simulink model "ELECTRIC_CIRCUIT_FINAL"  (R2018b)
settings: Solver=VariableStepAuto  StartTime=0.0  StopTime=6*10^-5  RelTol=1e-3
libraries: fl_lib x23, nesl_utility x14
settings Model: Creator=EmanuelCruvinel  LastModifiedBy=EmanuelCruvinel
settings SimscapeCC: SimscapeLogType=all

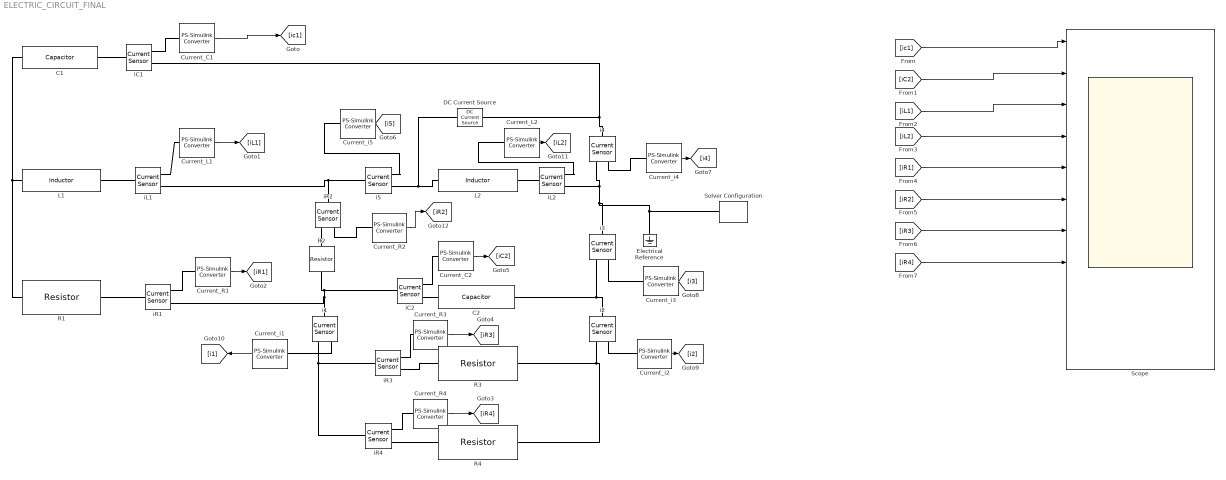
== system ELECTRIC_CIRCUIT_FINAL ==
  C1 : fl_lib/Electrical/Electrical Elements/Capacitor  c=1e-6 F  r=1e-6 Ohm  g=0 1/Ohm  i_specify=off  i_priority=None  i=0 A  i_nominal_specify=off  i_nominal_unit=A  i_nominal_value=1  v_specify=off  v_priority=None  v=0 V  v_nominal_specify=off  v_nominal_unit=V  v_nominal_value=1  vc_specify=off  vc_priority=High  vc=0 V  vc_nominal_specify=off  vc_nominal_unit=V  vc_nominal_value=1
  C2 : fl_lib/Electrical/Electrical Elements/Capacitor  c=1e-6 F  r=1e-6 Ohm  g=0 1/Ohm  i_specify=off  i_priority=None  i=0 A  i_nominal_specify=off  i_nominal_unit=A  i_nominal_value=1  v_specify=off  v_priority=None  v=0 V  v_nominal_specify=off  v_nominal_unit=V  v_nominal_value=1  vc_specify=off  vc_priority=High  vc=0 V  vc_nominal_specify=off  vc_nominal_unit=V  vc_nominal_value=1
  Current_C1 : nesl_utility/PS-Simulink Converter  PhysicalDomain=network_engine_domain  SubClassName=ps_output  LeftPortType=input  RightPortType=output  PseudoPeriodic=off  Frequencies=[]  Unit=1  AffineConversion=off
  Current_C2 : nesl_utility/PS-Simulink Converter  PhysicalDomain=network_engine_domain  SubClassName=ps_output  LeftPortType=input  RightPortType=output  PseudoPeriodic=off  Frequencies=[]  Unit=1  AffineConversion=off
  Current_L1 : nesl_utility/PS-Simulink Converter  PhysicalDomain=network_engine_domain  SubClassName=ps_output  LeftPortType=input  RightPortType=output  PseudoPeriodic=off  Frequencies=[]  Unit=1  AffineConversion=off
  Current_L2 : nesl_utility/PS-Simulink Converter  PhysicalDomain=network_engine_domain  SubClassName=ps_output  LeftPortType=input  RightPortType=output  PseudoPeriodic=off  Frequencies=[]  Unit=1  AffineConversion=off
  Current_R{1..4} (4 alike) : nesl_utility/PS-Simulink Converter  PhysicalDomain=network_engine_domain  SubClassName=ps_output  LeftPortType=input  RightPortType=output  PseudoPeriodic=off  Frequencies=[]  Unit=1  AffineConversion=off
  Current_i{1..5} (5 alike) : nesl_utility/PS-Simulink Converter  PhysicalDomain=network_engine_domain  SubClassName=ps_output  LeftPortType=input  RightPortType=output  PseudoPeriodic=off  Frequencies=[]  Unit=1  AffineConversion=off
  DC Current Source : fl_lib/Electrical/Electrical Sources/DC Current Source  i0=200 A
      settings: SourceProductName=Simscape  SourceProductBaseCode=SS
  Electrical Reference : fl_lib/Electrical/Electrical Elements/Electrical Reference
  L1 : fl_lib/Electrical/Electrical Elements/Inductor  l=1e-6 H  r=0 Ohm  g=1e-9 1/Ohm  i_specify=off  i_priority=None  i=0 A  i_nominal_specify=off  i_nominal_unit=A  i_nominal_value=1  v_specify=off  v_priority=None  v=0 V  v_nominal_specify=off  v_nominal_unit=V  v_nominal_value=1  i_L_specify=off  i_L_priority=High  i_L=0 A  i_L_nominal_specify=off  i_L_nominal_unit=A  i_L_nominal_value=1
  L2 : fl_lib/Electrical/Electrical Elements/Inductor  l=1e-6 H  r=0 Ohm  g=1e-9 1/Ohm  i_specify=off  i_priority=None  i=0 A  i_nominal_specify=off  i_nominal_unit=A  i_nominal_value=1  v_specify=off  v_priority=None  v=0 V  v_nominal_specify=off  v_nominal_unit=V  v_nominal_value=1  i_L_specify=off  i_L_priority=High  i_L=0 A  i_L_nominal_specify=off  i_L_nominal_unit=A  i_L_nominal_value=1
  R{1..4} (4 alike) : fl_lib/Electrical/Electrical Elements/Resistor  R=10 Ohm  i_specify=off  i_priority=None  i=0 A  i_nominal_specify=off  i_nominal_unit=A  i_nominal_value=1  v_specify=off  v_priority=None  v=0 V  v_nominal_specify=off  v_nominal_unit=V  v_nominal_value=1
      R1 settings: LogSimulationData=on
  Scope : Scope  NumInputPorts=11
  Solver Configuration : nesl_utility/Solver Configuration  PhysicalDomain=network_engine_domain  SubClassName=solver  LeftPortType=input  RightPortType=generic  Tones=[]  Harmonics=[]  SimulateNoise=off  Profile=off  UseLocalSampling=off  EnableSwitchedLinearOptims=on  FrequencyDomain=off  UseCCode=off  RelTol=0.001  AbsTol=1e-06  MinStep=1e-09  ToWorkspace=off  RevertToSquareIcSolve=off  NumHomotopyIterations=100  PhasorMode=off  PhasorModeNumHarmonics=1  DoDC=off  ResidualTolerance=1e-09  UseLocalSolver=off  LocalSolverChoice=NE_BACKWARD_EULER_ADVANCER  LocalSolverSampleTime=0.001  DoFixedCost=off  MaxNonlinIter=3  MaxModeIter=2  LinearAlgebra=auto  EquationFormulation=NE_TIME_EF  DelaysMemoryBudget=1024  AutomaticFiltering=on  FilteringTimeConstant=0.001  PartitionStorageMethod=AS_NEEDED  PartitionMemoryBudget=1024
  i{1..5} (5 alike) : fl_lib/Electrical/Electrical Sensors/Current Sensor
  iC1 : fl_lib/Electrical/Electrical Sensors/Current Sensor
  iC2 : fl_lib/Electrical/Electrical Sensors/Current Sensor
  iL1 : fl_lib/Electrical/Electrical Sensors/Current Sensor
  iL2 : fl_lib/Electrical/Electrical Sensors/Current Sensor
  iR{1..4} (4 alike) : fl_lib/Electrical/Electrical Sensors/Current Sensor
  wires:
  Current_C1/1 -> [ic1]
  [ic1] -> Scope/1
  Current_L1/1 -> [iL1]
  Current_R1/1 -> [iR1]
  Current_R4/1 -> [iR4]
  Current_R3/1 -> [iR3]
  Current_C2/1 -> [iC2]
  Current_i5/1 -> [i5]
  Current_i4/1 -> [i4]
  Current_i2/1 -> [i2]
  Current_i1/1 -> [i1]
  Current_L2/1 -> [iL2]
  [iC2] -> Scope/2
  [iL1] -> Scope/3
  [iL2] -> Scope/4
  [iR1] -> Scope/5
  [iR2] -> Scope/6
  [iR3] -> Scope/7
  [iR4] -> Scope/8
  Current_R2/1 -> [iR2]
  connections:
  R2/RConn1 -- iC2/LConn1 -- i1/LConn1 -- iR1/RConn2
  DC Current Source/RConn1 -- iC1/RConn2 -- i4/LConn1
  i5/LConn1 -- iR2/LConn1 -- iL1/RConn2
  L1/LConn1 -- C1/LConn1 -- R1/LConn1
  i5/RConn2 -- DC Current Source/LConn1 -- L2/LConn1
  iC1/LConn1 -- C1/RConn1
  iL1/LConn1 -- L1/RConn1
  iR1/LConn1 -- R1/RConn1
  iR3/LConn1 -- i1/RConn2 -- iR4/LConn1
  iR3/RConn2 -- R3/LConn1
  iR4/RConn2 -- R4/LConn1
  R4/RConn1 -- i2/RConn2 -- R3/RConn1
  i2/LConn1 -- i3/RConn2 -- C2/RConn1
  Electrical Reference/LConn1 -- iL2/RConn2 -- i4/RConn2 -- i3/LConn1 -- Solver Configuration/RConn1
  iL2/LConn1 -- L2/RConn1
  iC2/RConn2 -- C2/LConn1
  iC1/RConn1 -- Current_C1/LConn1
  iL1/RConn1 -- Current_L1/LConn1
  iR1/RConn1 -- Current_R1/LConn1
  Current_i1/LConn1 -- i1/RConn1
  iR4/RConn1 -- Current_R4/LConn1
  iR3/RConn1 -- Current_R3/LConn1
  iC2/RConn1 -- Current_C2/LConn1
  i5/RConn1 -- Current_i5/LConn1
  i4/RConn1 -- Current_i4/LConn1
  iL2/RConn1 -- Current_L2/LConn1
  i3/RConn1 -- Current_i3/LConn1
  i2/RConn1 -- Current_i2/LConn1
  iR2/RConn2 -- R2/LConn1
  iR2/RConn1 -- Current_R2/LConn1
